simulink model "fig9_46"  (Simulink 7.0)
settings: Solver=ode45  SolverMode=SingleTasking  StartTime=0.0  StopTime=15.0  RelTol=1e-3  AbsTol=1e-6
settings Model: Creator=abbas  LastModifiedBy=abbas  ExtModeTrigMode=oneshot  ExtModeArmWhenConnect=off  ExtModeAutoUpdateStatusClock=off
settings DataIOCC: LimitDataPoints=off
settings OptimizationCC: BlockReduction=off  BooleanDataType=off  InlineInvariantSignals=on
settings DebuggingCC: SaveWithParameterizedLinksMsg=none  SignalResolutionControl=TryResolveAllWithWarning  SolverPrmCheckMsg=none  MultiTaskDSMMsg=warning  MultiTaskCondExecSysMsg=none  StrictBusMsg=None
settings HardwareCC: TargetUnknown=on
settings RTWCC: IncludeERTFirstTime=on
settings GRTTargetCC: TargetFcnLib=ansi_tfl_tmw.mat  ModelReferenceCompliant=off  CompOptLevelCompliant=off  MatFileLogging=off

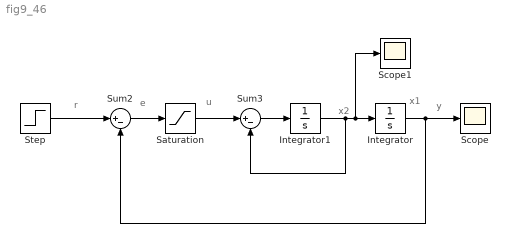
== system fig9_46 ==
  note: r
  note: e
  note: u
  note: x2
  note: x1
  note: y
  Integrator : Integrator
  Integrator1 : Integrator
  Saturation : Saturate
  Scope : Scope
      settings: TickLabels=on  DataFormat=Array
  Scope1 : Scope
      settings: TickLabels=on  DataFormat=Array
  Step : Step  Time=0  SampleTime=0.1
  Sum2 : Sum  Inputs=|+-  OutDataType=sfix(16)  OutScaling=2^0  SaturateOnIntegerOverflow=on  InputSameDT=on
  Sum3 : Sum  Inputs=|+-  OutDataType=sfix(16)  OutScaling=2^0  SaturateOnIntegerOverflow=on  InputSameDT=on
  wires:
  Sum2/1 -> Saturation/1
  Sum3/1 -> Integrator1/1
  Integrator/1 -> Scope/1, Sum2/2
  Step/1 -> Sum2/1
  Integrator1/1 -> Sum3/2, Integrator/1, Scope1/1
  Saturation/1 -> Sum3/1
